simulink model "test_pkt_pack_new_packet_format"  (Simulink 7.0)
settings: Solver=ode45  StartTime=0.0  StopTime=10000  RelTol=1e-3
libraries: xbsIndex_r4 x101, xps_library x3, casper_library x2
settings Model: Creator=Jason Manley  LastModifiedBy=dsp
settings DebuggingCC: SaveWithParameterizedLinksMsg=none  SignalResolutionControl=TryResolveAllWithWarning  MultiTaskDSMMsg=warning  MultiTaskCondExecSysMsg=none  StrictBusMsg=None
settings RTWCC: IncludeERTFirstTime=on
settings GRTTargetCC: TargetFcnLib=ansi_tfl_tmw.mat

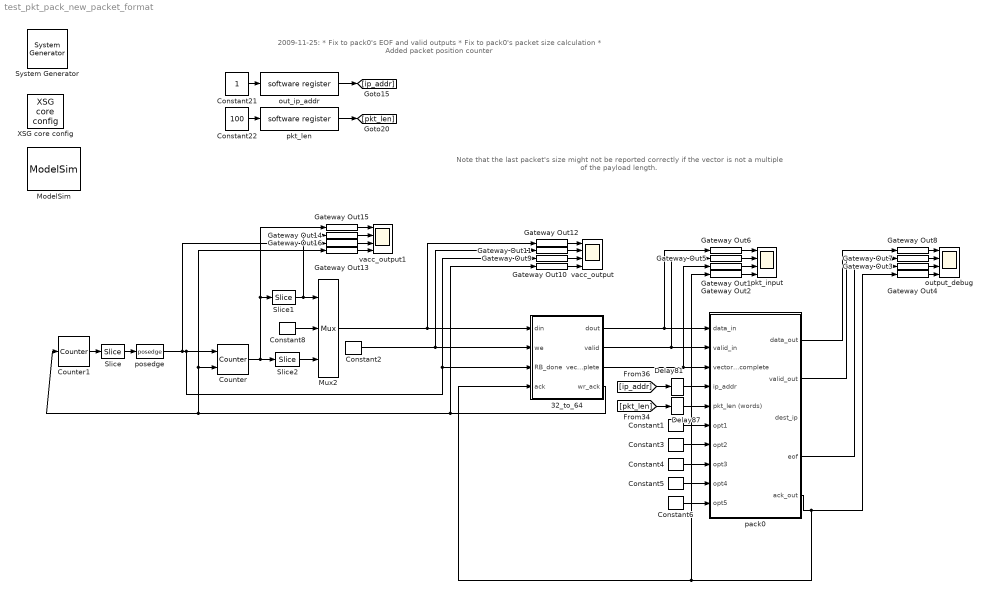
== system test_pkt_pack_new_packet_format ==
  note: 2009-11-25:
      |  * Fix to pack0's EOF and valid outputs
      |  * Fix to pack0's packet size calculation
      |  * Added packet position counter
  note: Note that the last packet's size might not be
      | reported correctly if the vector is not a multiple of the payload length.
  " System Generator" : xbsIndex_r4/ System Generator  Tag=genX  SystemSampleTime=-1  xilinxfamily=Virtex2P  part=xc2vp70  speed=-7  package=ff1704  synthesis_tool=XST  clock_wrapper=Clock Enables  directory=./test_d_v_p/sysgen  testbench=off  simulink_period=1  sysclk_period=4.878  dcm_input_clock_period=100  incr_netlist=off  trim_vbits=Everywhere in SubSystem  dbl_ovrd=According to Block Masks  core_generation=According to Block Masks  run_coregen=off  deprecated_control=off  eval_field=0  block_type=sysgen
      settings: block_version=10.1.3
  32_to_64 : Subsystem
  Constant1 : xbsIndex_r4/Constant  arith_type=Unsigned  const=101  n_bits=64  bin_pt=0  explicit_period=on  period=1  equ=P=C  opselect=C  inp2=PCIN>>17  opr=+  inp1=P  carry=CIN  dbl_ovrd=off  block_type=constant
  Constant2 : xbsIndex_r4/Constant  arith_type=Boolean  const=1  n_bits=3  bin_pt=0  explicit_period=on  period=1  equ=P=C  opselect=C  inp2=PCIN>>17  opr=+  inp1=P  carry=CIN  dbl_ovrd=off  block_type=constant
  Constant21 : Constant  OutDataType=sfix(16)  OutScaling=2^0
  Constant22 : Constant  Value=100  OutDataType=sfix(16)  OutScaling=2^0
  Constant3 : xbsIndex_r4/Constant  arith_type=Unsigned  const=102  n_bits=64  bin_pt=0  explicit_period=on  period=1  equ=P=C  opselect=C  inp2=PCIN>>17  opr=+  inp1=P  carry=CIN  dbl_ovrd=off  block_type=constant
  Constant4 : xbsIndex_r4/Constant  arith_type=Unsigned  const=103  n_bits=64  bin_pt=0  explicit_period=on  period=1  equ=P=C  opselect=C  inp2=PCIN>>17  opr=+  inp1=P  carry=CIN  dbl_ovrd=off  block_type=constant
  Constant5 : xbsIndex_r4/Constant  arith_type=Unsigned  const=104  n_bits=64  bin_pt=0  explicit_period=on  period=1  equ=P=C  opselect=C  inp2=PCIN>>17  opr=+  inp1=P  carry=CIN  dbl_ovrd=off  block_type=constant
  Constant6 : xbsIndex_r4/Constant  arith_type=Unsigned  const=105  n_bits=64  bin_pt=0  explicit_period=on  period=1  equ=P=C  opselect=C  inp2=PCIN>>17  opr=+  inp1=P  carry=CIN  dbl_ovrd=off  block_type=constant
  Constant8 : xbsIndex_r4/Constant  arith_type=Unsigned  const=0  n_bits=32  bin_pt=0  explicit_period=on  period=1  equ=P=C  opselect=C  inp2=PCIN>>17  opr=+  inp1=P  carry=CIN  dbl_ovrd=off  block_type=constant
  Counter : xbsIndex_r4/Counter  cnt_type=Free Running  cnt_to=Inf  operation=Up  start_count=0  cnt_by_val=1  arith_type=Unsigned  n_bits=33  bin_pt=0  load_pin=off  rst=on  en=on  explicit_period=on  period=1  dbl_ovrd=off  use_behavioral_HDL=off  use_rpm=off  implementation=Fabric  block_type=counter
  Counter1 : xbsIndex_r4/Counter  cnt_type=Free Running  cnt_to=Inf  operation=Up  start_count=0  cnt_by_val=1  arith_type=Unsigned  n_bits=14  bin_pt=0  load_pin=off  rst=off  en=on  explicit_period=on  period=1  dbl_ovrd=off  use_behavioral_HDL=off  use_rpm=off  implementation=Fabric  block_type=counter
  Delay81 : xbsIndex_r4/Delay  en=off  latency=5  dbl_ovrd=off  reg_retiming=on  block_type=delay
      settings: xl_area=[0, 0, 0, 0, 0, 0, 0]
  Delay87 : xbsIndex_r4/Delay  en=off  latency=5  dbl_ovrd=off  reg_retiming=on  block_type=delay
      settings: xl_area=[0, 0, 0, 0, 0, 0, 0]
  Gateway Out{1..16} (16 alike) : xbsIndex_r4/Gateway Out  hdl_port=on  timing_constraint=None  locs_specified=off  LOCs={}  block_type=gatewayout
      settings: infoedit="Gateway out block.  Converts Xilinx fixed point inputs into ouputs of type Simulink integer, double, or fixed point.<P><P>Hardware notes:  In hardware these blocks become top level output ports or are discarded, depending on how they are configured."  xl_area=[0, 0, 0, 0, 0, 0, 0]  block_version=10.1.3
  ModelSim : xbsIndex_r4/ModelSim  dir=./modelsim  waveform=on  leave_open=on  skip_compile=off  use_unisim=off  custom_scripts=off  startup_timeout=40  block_type=hdlcosim
      settings: infoedit="Allow other blocks to schedule HDL co-simulation tasks.<P><P>Note that selecting \"Skip compilation\" when inappropriate can cause simulation errors and failures. Please refer to the block help for details."  block_version=10.1.3
  Mux2 : xbsIndex_r4/Mux  inputs=2  en=off  latency=0  precision=Full  arith_type="Signed  (2's comp)"  n_bits=8  bin_pt=2  quantization=Truncate  overflow=Wrap  dbl_ovrd=off  block_type=mux
      settings: xl_area=[0, 0, 0, 0, 0, 0, 0]
  Slice : xbsIndex_r4/Slice  nbits=1  boolean_output=on  mode=Lower Bit Location + Width  bit1=0  base1=MSB of Input  bit0=10  base0=LSB of Input  dbl_ovrd=off  block_type=slice
      settings: infoedit="Extracts a given range of bits from each input sample and presents it at the output.  The output type is ordinarily unsigned with binary point at zero, but can be Boolean when the slice is one bit wide.<P><P>Hardware notes: In hardware this block costs nothing."  block_version=10.1.3
  Slice1 : xbsIndex_r4/Slice  nbits=1  boolean_output=on  mode=Lower Bit Location + Width  bit1=0  base1=MSB of Input  bit0=0  base0=LSB of Input  dbl_ovrd=off  block_type=slice
      settings: infoedit="Extracts a given range of bits from each input sample and presents it at the output.  The output type is ordinarily unsigned with binary point at zero, but can be Boolean when the slice is one bit wide.<P><P>Hardware notes: In hardware this block costs nothing."  block_version=10.1.3
  Slice2 : xbsIndex_r4/Slice  nbits=32  boolean_output=off  mode=Lower Bit Location + Width  bit1=0  base1=MSB of Input  bit0=1  base0=LSB of Input  dbl_ovrd=off  block_type=slice
      settings: infoedit="Extracts a given range of bits from each input sample and presents it at the output.  The output type is ordinarily unsigned with binary point at zero, but can be Boolean when the slice is one bit wide.<P><P>Hardware notes: In hardware this block costs nothing."  block_version=10.1.3
  XSG core config : xps_library/XSG core config  Tag=xps:xsg  SystemSampleTime=-1  hw_sys=BEE2_usr  ibob_linux=off  clk_src=sys_clk  iBOB_clk_src=sys_clk  BEE2_ctrl_clk_src=sys_clk  BEE2_usr_clk_src=sys_clk  ROACH_clk_src=sys_clk  CORR_clk_src=sys_clk  gpio_clk_io_group=iBOB:sma  gpio_clk_bit_index=0  clk_rate=100  sample_period=1  synthesis_tool=XST  mpc_type=powerpc405
  out_ip_addr : xps_library/software register  Tag=xps:sw_reg  SystemSampleTime=-1  io_dir=From Processor  arith_type=Unsigned  bitwidth=32  bin_pt=0  sample_period=1  gw_name=test_pkt_pack_new_packet_format_out_ip_addr_user_data_out
      link override test_d_v_p_10_1_new_packet_format_out_ip_addr_user_data_out: arith_type=Unsigned  n_bits=32  bin_pt=0  period=1
      link override test_pkt_pack_new_packet_format_out_ip_addr_user_data_out: arith_type=Unsigned  n_bits=32  bin_pt=0  period=1
  output_debug : Scope  NumInputPorts=4
      settings: YMin=-1~0~0~0  YMax=1~150~1~1  SaveName=ScopeData2
  pack0 : Subsystem  mask(pkt_pack_mask){vector_len=1024, magic_id=hex2dec('4b52'), ver_id=1}
      mask prompts: vector_len "vector length"; magic_id "Magic Identifier"; ver_id "Version Identifier"
      mask help:
      | This block generates packets from a datastream.
      |
      | Packets are created with a fixed header followed by a user-specified number of 64-bit options.
      |
      | Requires a 64-bit data stream.
      |
      | See the documentation for further details.
      mask init:
      | vector_bits = ceil(log2(vector_len));
  pkt_input : Scope  NumInputPorts=4
      settings: YMin=-1~0~0~0  YMax=1~150~1~1
  pkt_len : xps_library/software register  Tag=xps:sw_reg  SystemSampleTime=-1  io_dir=From Processor  arith_type=Unsigned  bitwidth=32  bin_pt=0  sample_period=1  gw_name=test_pkt_pack_new_packet_format_pkt_len_user_data_out
      link override test_d_v_p_10_1_new_packet_format_pkt_len_user_data_out: arith_type=Unsigned  n_bits=32  bin_pt=0  period=1
      link override test_pkt_pack_new_packet_format_pkt_len_user_data_out: arith_type=Unsigned  n_bits=32  bin_pt=0  period=1
  posedge : casper_library/Misc/posedge  Tag=Rising Edge Detector  SystemSampleTime=-1
  vacc_output : Scope  NumInputPorts=4
      settings: TimeRange=10000  YMin=0~0~0~0  YMax=1200~2~1~2  SaveName=ScopeData3
  vacc_output1 : Scope  NumInputPorts=4
      settings: YMin=-1~0~0~0  YMax=1~150~1~1  SaveName=ScopeData4
  wires:
  [ip_addr] -> Delay81/1
  [pkt_len] -> Delay87/1
  Delay81/1 -> pack0/4(ip_addr)
  Delay87/1 -> pack0/5(pkt_len (words))
  Constant22/1 -> pkt_len/1
  Constant21/1 -> out_ip_addr/1
  out_ip_addr/1 -> [ip_addr]
  pkt_len/1 -> [pkt_len]
  pack0/4(eof) -> Gateway Out3/1
  Counter1/1 -> Slice/1
  posedge/1 -> Gateway Out16/1, Counter/1, Gateway Out9/1, 32_to_64/3(RB_done)
  pack0/5(ack_out) -> Gateway Out4/1, Gateway Out2/1, 32_to_64/4(ack)
  Slice/1 -> posedge/1
  Gateway Out6/1 -> pkt_input/1
  Gateway Out5/1 -> pkt_input/2
  Gateway Out1/1 -> pkt_input/3
  Gateway Out2/1 -> pkt_input/4
  Constant1/1 -> pack0/6(opt1)
  Constant3/1 -> pack0/7(opt2)
  Constant4/1 -> pack0/8(opt3)
  Constant5/1 -> pack0/9(opt4)
  Constant6/1 -> pack0/10(opt5)
  Gateway Out8/1 -> output_debug/1
  Gateway Out7/1 -> output_debug/2
  Gateway Out3/1 -> output_debug/3
  Gateway Out4/1 -> output_debug/4
  pack0/1(data_out) -> Gateway Out8/1
  pack0/2(valid_out) -> Gateway Out7/1
  Counter/1 -> Slice2/1, Slice1/1, Gateway Out15/1
  32_to_64/1(dout) -> Gateway Out6/1, pack0/1(data_in)
  32_to_64/2(valid) -> Gateway Out5/1, pack0/2(valid_in)
  32_to_64/3(vector_complete) -> Gateway Out1/1, pack0/3(vector_complete)
  Constant8/1 -> Mux2/2
  Slice1/1 -> Mux2/1, Gateway Out14/1
  Slice2/1 -> Mux2/3
  Gateway Out15/1 -> vacc_output1/1
  Gateway Out14/1 -> vacc_output1/2
  Gateway Out16/1 -> vacc_output1/3
  Gateway Out13/1 -> vacc_output1/4
  Constant2/1 -> Gateway Out11/1, 32_to_64/2(we)
  Mux2/1 -> Gateway Out12/1, 32_to_64/1(din)
  Gateway Out12/1 -> vacc_output/1
  Gateway Out11/1 -> vacc_output/2
  Gateway Out9/1 -> vacc_output/3
  Gateway Out10/1 -> vacc_output/4
  32_to_64/4(wr_ack) -> Gateway Out10/1, Counter/2, Gateway Out13/1, Counter1/1

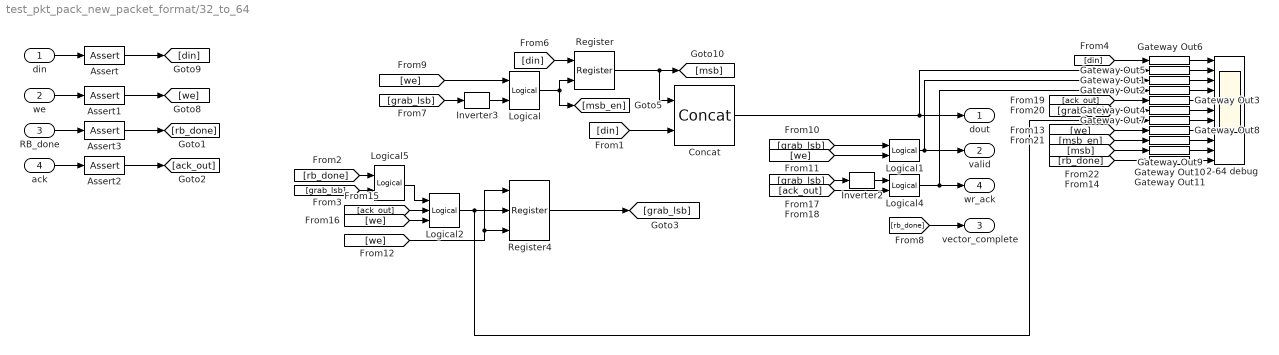
== system test_pkt_pack_new_packet_format/32_to_64 ==
  din : Inport  OutDataType=sfix(16)  OutScaling=2^0
  we : Inport  Port=2  OutDataType=sfix(16)  OutScaling=2^0
  RB_done : Inport  Port=3  OutDataType=sfix(16)  OutScaling=2^0
  ack : Inport  Port=4  OutDataType=sfix(16)  OutScaling=2^0
  32-64 debug : Scope  NumInputPorts=11
      settings: YMin=-1~0~0~0~-5~-5~-5~-5~-5~-5~-5  YMax=1~150~1~1~5~5~5~5~5~5~5  SaveName=ScopeData5
  Assert : xbsIndex_r4/Assert  assert_type=on  type_source=Explicitly  arith_type=Unsigned  n_bits=32  bin_pt=0  assert_rate=off  rate_source=Explicitly  period=1  output_port=on  block_type=assert
      settings: infoedit=Asserts a user-defined sample rate and/or type on a signal.<P><P>Hardware notes: In hardware this block costs nothing.  block_version=10.1.3
  Assert1 : xbsIndex_r4/Assert  assert_type=on  type_source=Explicitly  arith_type=Boolean  n_bits=32  bin_pt=0  assert_rate=off  rate_source=Explicitly  period=1  output_port=on  block_type=assert
      settings: infoedit=Asserts a user-defined sample rate and/or type on a signal.<P><P>Hardware notes: In hardware this block costs nothing.  block_version=10.1.3
  Assert2 : xbsIndex_r4/Assert  assert_type=on  type_source=Explicitly  arith_type=Boolean  n_bits=32  bin_pt=0  assert_rate=off  rate_source=Explicitly  period=1  output_port=on  block_type=assert
      settings: infoedit=Asserts a user-defined sample rate and/or type on a signal.<P><P>Hardware notes: In hardware this block costs nothing.  block_version=10.1.3
  Assert3 : xbsIndex_r4/Assert  assert_type=on  type_source=Explicitly  arith_type=Boolean  n_bits=32  bin_pt=0  assert_rate=off  rate_source=Explicitly  period=1  output_port=on  block_type=assert
      settings: infoedit=Asserts a user-defined sample rate and/or type on a signal.<P><P>Hardware notes: In hardware this block costs nothing.  block_version=10.1.3
  Concat : xbsIndex_r4/Concat  num_inputs=2  dbl_ovrd=off  block_type=concat
      settings: block_version=10.1.3
  Gateway Out{1..11} (11 alike) : xbsIndex_r4/Gateway Out  hdl_port=on  timing_constraint=None  locs_specified=off  LOCs={}  block_type=gatewayout
      settings: infoedit="Gateway out block.  Converts Xilinx fixed point inputs into ouputs of type Simulink integer, double, or fixed point.<P><P>Hardware notes:  In hardware these blocks become top level output ports or are discarded, depending on how they are configured."  xl_area=[0, 0, 0, 0, 0, 0, 0]  block_version=10.1.3
  Inverter2 : xbsIndex_r4/Inverter  en=off  latency=0  dbl_ovrd=off  block_type=inv
  Inverter3 : xbsIndex_r4/Inverter  en=off  latency=0  dbl_ovrd=off  block_type=inv
  Logical : xbsIndex_r4/Logical  logical_function=AND  inputs=2  en=off  latency=0  precision=Full  arith_type=Unsigned  n_bits=16  bin_pt=0  align_bp=on  dbl_ovrd=off  block_type=logical
  Logical1 : xbsIndex_r4/Logical  logical_function=AND  inputs=2  en=off  latency=0  precision=Full  arith_type=Unsigned  n_bits=16  bin_pt=0  align_bp=on  dbl_ovrd=off  block_type=logical
  Logical2 : xbsIndex_r4/Logical  logical_function=AND  inputs=3  en=off  latency=0  precision=Full  arith_type=Unsigned  n_bits=16  bin_pt=0  align_bp=on  dbl_ovrd=off  block_type=logical
  Logical4 : xbsIndex_r4/Logical  logical_function=OR  inputs=2  en=off  latency=0  precision=Full  arith_type=Unsigned  n_bits=16  bin_pt=0  align_bp=on  dbl_ovrd=off  block_type=logical
  Logical5 : xbsIndex_r4/Logical  logical_function=OR  inputs=2  en=off  latency=0  precision=Full  arith_type=Unsigned  n_bits=16  bin_pt=0  align_bp=on  dbl_ovrd=off  block_type=logical
  Register : xbsIndex_r4/Register  init=0  rst=off  en=on  dbl_ovrd=off  block_type=register
  Register4 : xbsIndex_r4/Register  init=0  rst=on  en=on  dbl_ovrd=off  block_type=register
  dout : Outport  OutDataType=sfix(16)  OutScaling=2^0
  valid : Outport  Port=2  OutDataType=sfix(16)  OutScaling=2^0
  vector_complete : Outport  Port=3  OutDataType=sfix(16)  OutScaling=2^0
  wr_ack : Outport  Port=4  OutDataType=sfix(16)  OutScaling=2^0
  wires:
  din/1 -> Assert/1
  ack/1 -> Assert2/1
  we/1 -> Assert1/1
  Assert/1 -> [din]
  Assert1/1 -> [we]
  Assert2/1 -> [ack_out]
  [din] -> Register/1
  Register/1 -> Concat/1, [msb]
  [din] -> Concat/2
  Logical4/1 -> wr_ack/1, Gateway Out2/1
  Logical1/1 -> valid/1, Gateway Out1/1
  Logical/1 -> Register/2, [msb_en]
  RB_done/1 -> Assert3/1
  Assert3/1 -> [rb_done]
  [rb_done] -> vector_complete/1
  Concat/1 -> dout/1, Gateway Out5/1
  Register4/1 -> [grab_lsb]
  [grab_lsb] -> Inverter3/1
  [we] -> Logical/1
  [grab_lsb] -> Inverter2/1
  [ack_out] -> Logical4/2
  Gateway Out6/1 -> 32-64 debug/1
  Gateway Out5/1 -> 32-64 debug/2
  Gateway Out1/1 -> 32-64 debug/3
  Gateway Out2/1 -> 32-64 debug/4
  [din] -> Gateway Out6/1
  [ack_out] -> Gateway Out3/1
  [grab_lsb] -> Gateway Out4/1
  Gateway Out3/1 -> 32-64 debug/5
  Gateway Out4/1 -> 32-64 debug/6
  Gateway Out7/1 -> 32-64 debug/7
  Gateway Out8/1 -> 32-64 debug/8
  Gateway Out9/1 -> 32-64 debug/9
  Gateway Out10/1 -> 32-64 debug/10
  [we] -> Gateway Out8/1
  [msb_en] -> Gateway Out9/1
  [msb] -> Gateway Out10/1
  [we] -> Logical1/2
  [grab_lsb] -> Logical1/1
  Inverter2/1 -> Logical4/1
  Inverter3/1 -> Logical/2
  [rb_done] -> Gateway Out11/1
  Gateway Out11/1 -> 32-64 debug/11
  Logical5/1 -> Logical2/1
  [ack_out] -> Logical2/2
  [we] -> Logical2/3
  [rb_done] -> Logical5/1
  Logical2/1 -> Register4/2, Gateway Out7/1
  [grab_lsb] -> Logical5/2
  [we] -> Register4/3, Register4/1

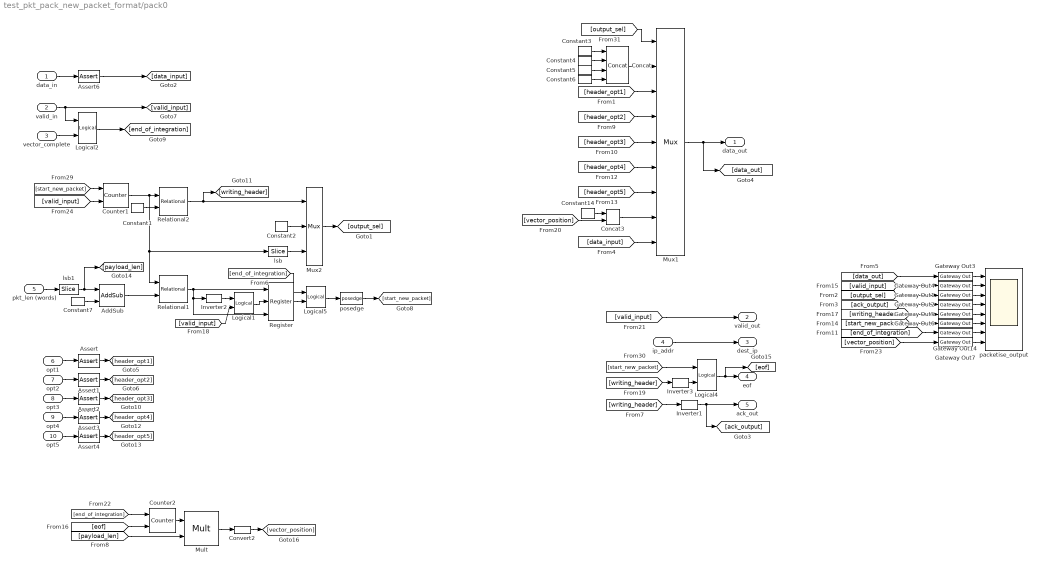
== system test_pkt_pack_new_packet_format/pack0 ==
  data_in : Inport  OutDataType=sfix(16)  OutScaling=2^0
  valid_in : Inport  Port=2  OutDataType=sfix(16)  OutScaling=2^0
  vector_complete : Inport  Port=3  OutDataType=sfix(16)  OutScaling=2^0
  ip_addr : Inport  Port=4  OutDataType=sfix(16)  OutScaling=2^0
  pkt_len (words) : Inport  Port=5  OutDataType=sfix(16)  OutScaling=2^0
  opt1 : Inport  Port=6  OutDataType=sfix(16)  OutScaling=2^0
  opt2 : Inport  Port=7  OutDataType=sfix(16)  OutScaling=2^0
  opt3 : Inport  Port=8  OutDataType=sfix(16)  OutScaling=2^0
  opt4 : Inport  Port=9  OutDataType=sfix(16)  OutScaling=2^0
  opt5 : Inport  Port=10  OutDataType=sfix(16)  OutScaling=2^0
  AddSub : xbsIndex_r4/AddSub  mode=Addition  use_carryin=off  use_carryout=off  en=off  latency=0  precision=Full  arith_type=Unsigned  n_bits=16  bin_pt=14  quantization=Truncate  overflow=Wrap  dbl_ovrd=off  use_behavioral_HDL=off  pipelined=off  use_rpm=on  hw_selection=Fabric  block_type=addsub
      settings: block_version=10.1.3
  Assert{,1..4,6} (6 alike) : xbsIndex_r4/Assert  assert_type=on  type_source=Explicitly  arith_type=Unsigned  n_bits=64  bin_pt=0  assert_rate=off  rate_source=Explicitly  period=1  output_port=on  block_type=assert
      settings: infoedit=Asserts a user-defined sample rate and/or type on a signal.<P><P>Hardware notes: In hardware this block costs nothing.  block_version=10.1.3
  Concat : xbsIndex_r4/Concat  num_inputs=4  dbl_ovrd=off  block_type=concat
      settings: block_version=10.1.3
  Concat3 : xbsIndex_r4/Concat  num_inputs=2  dbl_ovrd=off  block_type=concat
      settings: block_version=10.1.3
  Constant1 : xbsIndex_r4/Constant  arith_type=Unsigned  const=7  n_bits=3  bin_pt=0  explicit_period=on  period=1  equ=P=C  opselect=C  inp2=PCIN>>17  opr=+  inp1=P  carry=CIN  dbl_ovrd=off  block_type=constant
  Constant14 : xbsIndex_r4/Constant  arith_type=Unsigned  const=5  n_bits=16  bin_pt=0  explicit_period=on  period=1  equ=P=C  opselect=C  inp2=PCIN>>17  opr=+  inp1=P  carry=CIN  dbl_ovrd=off  block_type=constant
  Constant2 : xbsIndex_r4/Constant  arith_type=Unsigned  const=7  n_bits=3  bin_pt=0  explicit_period=on  period=1  equ=P=C  opselect=C  inp2=PCIN>>17  opr=+  inp1=P  carry=CIN  dbl_ovrd=off  block_type=constant
  Constant3 : xbsIndex_r4/Constant  arith_type=Unsigned  const=magic_id  n_bits=16  bin_pt=0  explicit_period=on  period=1  equ=P=C  opselect=C  inp2=PCIN>>17  opr=+  inp1=P  carry=CIN  dbl_ovrd=off  block_type=constant
  Constant4 : xbsIndex_r4/Constant  arith_type=Unsigned  const=ver_id  n_bits=16  bin_pt=0  explicit_period=on  period=1  equ=P=C  opselect=C  inp2=PCIN>>17  opr=+  inp1=P  carry=CIN  dbl_ovrd=off  block_type=constant
  Constant5 : xbsIndex_r4/Constant  arith_type=Unsigned  const=0  n_bits=16  bin_pt=0  explicit_period=on  period=1  equ=P=C  opselect=C  inp2=PCIN>>17  opr=+  inp1=P  carry=CIN  dbl_ovrd=off  block_type=constant
  Constant6 : xbsIndex_r4/Constant  arith_type=Unsigned  const=6  n_bits=16  bin_pt=0  explicit_period=on  period=1  equ=P=C  opselect=C  inp2=PCIN>>17  opr=+  inp1=P  carry=CIN  dbl_ovrd=off  block_type=constant
  Constant7 : xbsIndex_r4/Constant  arith_type=Unsigned  const=7-1  n_bits=3  bin_pt=0  explicit_period=on  period=1  equ=P=C  opselect=C  inp2=PCIN>>17  opr=+  inp1=P  carry=CIN  dbl_ovrd=off  block_type=constant
  Convert2 : xbsIndex_r4/Convert  arith_type=Unsigned  n_bits=48  bin_pt=0  quantization=Truncate  overflow=Wrap  latency=0  dbl_ovrd=off  pipeline=off  block_type=convert
      settings: block_version=10.1.3
  Counter1 : xbsIndex_r4/Counter  cnt_type=Free Running  cnt_to=1023  operation=Up  start_count=0  cnt_by_val=1  arith_type=Unsigned  n_bits=15  bin_pt=0  load_pin=off  rst=on  en=on  explicit_period=on  period=1  dbl_ovrd=off  use_behavioral_HDL=off  use_rpm=on  implementation=Fabric  block_type=counter
      settings: xl_area=[0, 0, 0, 0, 0, 0, 0]
  Counter2 : xbsIndex_r4/Counter  cnt_type=Free Running  cnt_to=1023  operation=Up  start_count=0  cnt_by_val=1  arith_type=Unsigned  n_bits=vector_bits+1  bin_pt=0  load_pin=off  rst=on  en=on  explicit_period=on  period=1  dbl_ovrd=off  use_behavioral_HDL=off  use_rpm=on  implementation=Fabric  block_type=counter
      settings: xl_area=[0, 0, 0, 0, 0, 0, 0]
  Gateway Out{1..7,14} (8 alike) : xbsIndex_r4/Gateway Out  hdl_port=on  timing_constraint=None  locs_specified=off  LOCs={}  block_type=gatewayout
      settings: infoedit="Gateway out block.  Converts Xilinx fixed point inputs into ouputs of type Simulink integer, double, or fixed point.<P><P>Hardware notes:  In hardware these blocks become top level output ports or are discarded, depending on how they are configured."  xl_area=[0, 0, 0, 0, 0, 0, 0]  block_version=10.1.3
  Inverter1 : xbsIndex_r4/Inverter  en=off  latency=0  dbl_ovrd=off  block_type=inv
      settings: xl_area=[0, 0, 0, 0, 0, 0, 0]
  Inverter2 : xbsIndex_r4/Inverter  en=off  latency=0  dbl_ovrd=off  block_type=inv
      settings: xl_area=[0, 0, 0, 0, 0, 0, 0]
  Inverter3 : xbsIndex_r4/Inverter  en=off  latency=0  dbl_ovrd=off  block_type=inv
      settings: xl_area=[0, 0, 0, 0, 0, 0, 0]
  Logical1 : xbsIndex_r4/Logical  logical_function=AND  inputs=2  en=off  latency=0  precision=Full  arith_type=Unsigned  n_bits=8  bin_pt=2  align_bp=on  dbl_ovrd=off  block_type=logical
      settings: xl_area=[0, 0, 0, 0, 0, 0, 0]
  Logical2 : xbsIndex_r4/Logical  logical_function=AND  inputs=2  en=off  latency=0  precision=Full  arith_type=Unsigned  n_bits=8  bin_pt=2  align_bp=on  dbl_ovrd=off  block_type=logical
      settings: xl_area=[0, 0, 0, 0, 0, 0, 0]
  Logical4 : xbsIndex_r4/Logical  logical_function=AND  inputs=2  en=off  latency=0  precision=Full  arith_type=Unsigned  n_bits=8  bin_pt=2  align_bp=on  dbl_ovrd=off  block_type=logical
      settings: xl_area=[0, 0, 0, 0, 0, 0, 0]
  Logical5 : xbsIndex_r4/Logical  logical_function=OR  inputs=2  en=off  latency=0  precision=Full  arith_type=Unsigned  n_bits=8  bin_pt=2  align_bp=on  dbl_ovrd=off  block_type=logical
      settings: xl_area=[0, 0, 0, 0, 0, 0, 0]
  Mult : xbsIndex_r4/Mult  precision=Full  arith_type="Signed  (2's comp)"  n_bits=16  bin_pt=14  quantization=Truncate  overflow=Wrap  en=off  latency=4  dbl_ovrd=off  use_behavioral_HDL=off  use_embedded=on  opt=Speed  optimum_pipeline=on  pipeline=on  use_rpm=on  placement_style=Triangular  block_type=mult
      settings: infoedit=Hardware notes: To use the internal pipeline stage of the dedicated multiplier you must select 'Pipeline for maximum performance'.  block_version=10.1.3
  Mux1 : xbsIndex_r4/Mux  inputs=8  en=off  latency=0  precision=Full  arith_type="Signed  (2's comp)"  n_bits=8  bin_pt=2  quantization=Truncate  overflow=Wrap  dbl_ovrd=off  block_type=mux
      settings: xl_area=[0, 0, 0, 0, 0, 0, 0]
  Mux2 : xbsIndex_r4/Mux  inputs=2  en=off  latency=0  precision=Full  arith_type="Signed  (2's comp)"  n_bits=8  bin_pt=2  quantization=Truncate  overflow=Wrap  dbl_ovrd=off  block_type=mux
      settings: xl_area=[0, 0, 0, 0, 0, 0, 0]
  Register : xbsIndex_r4/Register  init=0  rst=on  en=on  dbl_ovrd=off  block_type=register
  Relational1 : xbsIndex_r4/Relational  mode=a>=b  en=off  latency=0  dbl_ovrd=off  block_type=relational
      settings: xl_area=[0, 0, 0, 0, 0, 0, 0]  block_version=10.1.3
  Relational2 : xbsIndex_r4/Relational  mode=a<b  en=off  latency=0  dbl_ovrd=off  block_type=relational
      settings: xl_area=[0, 0, 0, 0, 0, 0, 0]  block_version=10.1.3
  lsb : xbsIndex_r4/Slice  nbits=3  boolean_output=off  mode=Lower Bit Location + Width  bit1=0  base1=MSB of Input  bit0=0  base0=LSB of Input  dbl_ovrd=off  block_type=slice
      settings: infoedit="Extracts a given range of bits from each input sample and presents it at the output.  The output type is ordinarily unsigned with binary point at zero, but can be Boolean when the slice is one bit wide.<P><P>Hardware notes: In hardware this block costs nothing."  block_version=10.1.3
  lsb1 : xbsIndex_r4/Slice  nbits=11  boolean_output=off  mode=Lower Bit Location + Width  bit1=0  base1=MSB of Input  bit0=0  base0=LSB of Input  dbl_ovrd=off  block_type=slice
      settings: infoedit="Extracts a given range of bits from each input sample and presents it at the output.  The output type is ordinarily unsigned with binary point at zero, but can be Boolean when the slice is one bit wide.<P><P>Hardware notes: In hardware this block costs nothing."  block_version=10.1.3
  packetise_output : Scope  NumInputPorts=8
      settings: YMin=0~0~0~0~0~0~0~-5  YMax=1200~1~5~1~100~1~1~5
  posedge : casper_library/Misc/posedge  Tag=Rising Edge Detector  SystemSampleTime=-1
  data_out : Outport  OutDataType=sfix(16)  OutScaling=2^0
  valid_out : Outport  Port=2  OutDataType=sfix(16)  OutScaling=2^0
  dest_ip : Outport  Port=3  OutDataType=sfix(16)  OutScaling=2^0
  eof : Outport  Port=4  OutDataType=sfix(16)  OutScaling=2^0
  ack_out : Outport  Port=5  OutDataType=sfix(16)  OutScaling=2^0
  wires:
  [ack_output] -> Gateway Out2/1
  [writing_header] -> Gateway Out5/1
  [end_of_integration] -> Gateway Out14/1
  Gateway Out14/1 -> packetise_output/7
  [valid_input] -> Gateway Out4/1
  [start_new_packet] -> Gateway Out6/1
  [end_of_integration] -> Logical5/1
  Gateway Out6/1 -> packetise_output/6
  Gateway Out5/1 -> packetise_output/5
  Gateway Out2/1 -> packetise_output/4
  Gateway Out1/1 -> packetise_output/3
  Gateway Out4/1 -> packetise_output/2
  Gateway Out3/1 -> packetise_output/1
  ip_addr/1 -> dest_ip/1
  valid_in/1 -> [valid_input], Logical2/1
  Mux1/1 -> data_out/1, [data_out]
  Logical5/1 -> posedge/1
  Counter1/1 -> Relational2/1, lsb/1, Relational1/1
  [valid_input] -> Counter1/2
  [start_new_packet] -> Counter1/1
  Relational2/1 -> [writing_header], Mux2/1
  Constant1/1 -> Relational2/2
  Mux2/1 -> [output_sel]
  [output_sel] -> Mux1/1
  [output_sel] -> Gateway Out1/1
  [data_out] -> Gateway Out3/1
  Inverter1/1 -> ack_out/1, [ack_output]
  [writing_header] -> Inverter1/1
  Logical2/1 -> [end_of_integration]
  vector_complete/1 -> Logical2/2
  data_in/1 -> Assert6/1
  opt1/1 -> Assert/1
  Assert/1 -> [header_opt1]
  Assert1/1 -> [header_opt2]
  Assert2/1 -> [header_opt3]
  Assert3/1 -> [header_opt4]
  Assert4/1 -> [header_opt5]
  opt2/1 -> Assert1/1
  opt3/1 -> Assert2/1
  opt4/1 -> Assert3/1
  opt5/1 -> Assert4/1
  [header_opt1] -> Mux1/3
  Concat/1 -> Mux1/2
  Constant3/1 -> Concat/1
  Constant4/1 -> Concat/2
  Constant5/1 -> Concat/3
  Constant6/1 -> Concat/4
  [data_input] -> Mux1/9
  [header_opt2] -> Mux1/4
  [header_opt3] -> Mux1/5
  [header_opt4] -> Mux1/6
  [header_opt5] -> Mux1/7
  Assert6/1 -> [data_input]
  Constant2/1 -> Mux2/2
  lsb/1 -> Mux2/3
  Relational1/1 -> Register/1, Register/3, Inverter2/1
  Register/1 -> Logical5/2
  [valid_input] -> Logical1/2
  posedge/1 -> [start_new_packet]
  Logical4/1 -> eof/1, [eof]
  [start_new_packet] -> Logical4/1
  Inverter3/1 -> Logical4/2
  [writing_header] -> Inverter3/1
  AddSub/1 -> Relational1/2
  pkt_len (words)/1 -> lsb1/1
  Constant7/1 -> AddSub/2
  lsb1/1 -> AddSub/1, [payload_len]
  Inverter2/1 -> Logical1/1
  Logical1/1 -> Register/2
  [valid_input] -> valid_out/1
  Constant14/1 -> Concat3/1
  [vector_position] -> Concat3/2
  Concat3/1 -> Mux1/8
  Counter2/1 -> Mult/1
  [eof] -> Counter2/2
  [payload_len] -> Mult/2
  Mult/1 -> Convert2/1
  Convert2/1 -> [vector_position]
  [end_of_integration] -> Counter2/1
  Gateway Out7/1 -> packetise_output/8
  [vector_position] -> Gateway Out7/1
